simulink model "Sistema_LTI_Equivalente"  (R2023b)
settings: Solver=VariableStepAuto  StartTime=0.0  StopTime=10.0  RelTol=1e-3
values from neighbouring files (symbols this model uses):
  lambda_m = 0.016    [parametros_proyecto2.m]
  Lq = 5.8e-3    (= 0.0058)    [parametros_proyecto2.m]
  r = 120    [parametros_proyecto2.m]
  Rs_ref = 1.02    [parametros_proyecto2.m]
  Rts_amb = 146.7    [parametros_proyecto2.m]
undefined symbols (not defined in the file or in its folder): cts, J_eq, magnitude, P_p
settings Model: Creator=ignab  LastModifiedBy=ignab

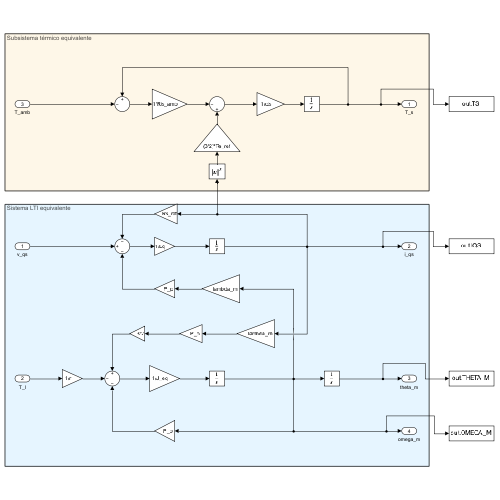
[thumbnail: Simulink's stored preview of the top-level diagram]
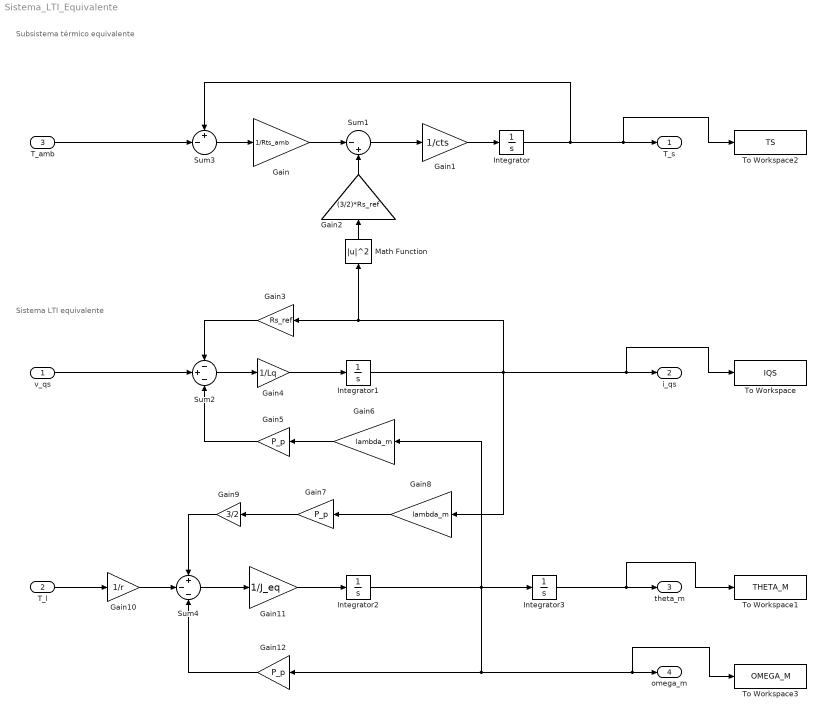
== system Sistema_LTI_Equivalente ==
  note: Sistema LTI equivalente
  note: Subsistema térmico equivalente
  v_qs : Inport
  T_l : Inport  Port=2
  T_amb : Inport  Port=3
  Gain : Gain  Gain=1/Rts_amb
  Gain1 : Gain  Gain=1/cts
  Gain10 : Gain  Gain=1/r
  Gain11 : Gain  Gain=1/J_eq
  Gain12 : Gain  Gain=P_p
  Gain2 : Gain  Gain=(3/2)*Rs_ref
  Gain3 : Gain  Gain=Rs_ref
  Gain4 : Gain  Gain=1/Lq
  Gain5 : Gain  Gain=P_p
  Gain6 : Gain  Gain=lambda_m
  Gain7 : Gain  Gain=P_p
  Gain8 : Gain  Gain=lambda_m
  Gain9 : Gain  Gain=3/2
  Integrator{,1..3} (4 alike) : Integrator
  Math Function : Math  Operator=magnitude^2
  Sum1 : Sum  Inputs=|-+
  Sum2 : Sum  Inputs=-+-
  Sum3 : Sum  Inputs=+-|
  Sum4 : Sum  Inputs=+--
  To Workspace : ToWorkspace  VariableName=IQS  SaveFormat=Timeseries  SampleTime=-1
      settings: Decimation=2
  To Workspace1 : ToWorkspace  VariableName=THETA_M  SaveFormat=Timeseries  SampleTime=-1
  To Workspace2 : ToWorkspace  VariableName=TS  SaveFormat=Timeseries  SampleTime=-1
  To Workspace3 : ToWorkspace  VariableName=OMEGA_M  SaveFormat=Timeseries  SampleTime=-1
  T_s : Outport
  i_qs : Outport  Port=2
  theta_m : Outport  Port=3
  omega_m : Outport  Port=4
  wires:
  T_amb/1 -> Sum3/2
  Sum3/1 -> Gain/1
  Gain2/1 -> Sum1/2
  Gain/1 -> Sum1/1
  Sum1/1 -> Gain1/1
  Gain1/1 -> Integrator/1
  Integrator/1 -> Sum3/1, To Workspace2/1, T_s/1
  Math Function/1 -> Gain2/1
  v_qs/1 -> Sum2/2
  Gain5/1 -> Sum2/3
  Gain3/1 -> Sum2/1
  Sum2/1 -> Gain4/1
  Gain4/1 -> Integrator1/1
  Gain6/1 -> Gain5/1
  Integrator1/1 -> Gain8/1, Math Function/1, Gain3/1, To Workspace/1, i_qs/1
  Gain8/1 -> Gain7/1
  Gain7/1 -> Gain9/1
  Gain9/1 -> Sum4/1
  Gain12/1 -> Sum4/3
  Sum4/1 -> Gain11/1
  Gain11/1 -> Integrator2/1
  Integrator3/1 -> To Workspace1/1, theta_m/1
  Integrator2/1 -> Integrator3/1, To Workspace3/1, omega_m/1, Gain12/1, Gain6/1
  Gain10/1 -> Sum4/2
  T_l/1 -> Gain10/1
